simulink model "SOGI_PLL_test"  (R2025a)
settings: Solver=FixedStepAuto  StartTime=0.0  StopTime=0.4  FixedStep=sample_time_s_d  RelTol=1e-3  EnableMultiTasking=on
undefined symbols (not defined in the file): DiscIntNeverNeededParam, filter_omega_sogi_a, filter_omega_sogi_b, filter_omega_sogi_init, filter_rms_out_a, filter_rms_out_b, filter_rms_out_init, grid_frequency_hz, k_rms, k_sogi_5th_hardmonic, pll_sat_max, pll_sat_min, SRF_PI_I, SRF_PI_P, Ts
libraries: simulink x2, spsAlphaBetaZerotodq0Lib x1, eeDiscretePi x1
settings Model: Creator=Masood  LastModifiedBy=li_hh
settings OptimizationCC: DefaultParameterBehavior=Inlined  UseDivisionForNetSlopeComputation=on  GainParamInheritBuiltInType=on  UseFloatMulNetSlope=on  InlineInvariantSignals=on  PassReuseOutputArgsAs=Individual arguments  ZeroExternalMemoryAtStartup=off  NoFixptDivByZeroProtection=on  EfficientFloat2IntCast=on  LifeSpan=1  MaxStackSize=2560  OptimizeBlockOrder=speed  DifferentSizesBufferReuse=on  EfficientTunableParamExpr=on
settings DebuggingCC: ParameterTunabilityLossMsg=error
settings HardwareCC: ProdBitPerPointer=32.0  ProdBitPerSizeT=32.0  ProdBitPerPtrDiffT=32.0  ProdLargestAtomicInteger=Long  ProdLargestAtomicFloat=Double  ProdWordSize=32.0  ProdLongLongMode=on  ProdHWDeviceType=ARM Compatible->ARM Cortex-M
settings SFSimCC: MATLABDynamicMemAlloc=off
settings RTWCC: SystemTargetFile=ert.tlc  TemplateMakefile=ert_default_tmf  Toolchain=Texas Instruments Code Composer Studio (ARM)  Description=Embedded Coder
settings CodeAppCC: ForceParamTrailComments=on  IgnoreCustomStorageClasses=off  OperatorAnnotations=on  SimulinkDataObjDesc=on  SFDataObjDesc=on  CustomSymbolStrGlobalVar=rt$N$M  CustomSymbolStrType=$N$M  CustomSymbolStrFcn=$N$M$F  CustomSymbolStrMacro=$N$M  InsertBlockDesc=on
settings ERTTargetCC: ExtModeTransport=3.0  ERTCustomFileTemplate=example_file_process.tlc  ERTFilePackagingFormat=CompactWithDataFile  IncludeMdlTerminateFcn=off  CombineSignalStateStructs=on  CodeInterfacePackaging=Reusable function  SupportComplex=off  SupportContinuousTime=on

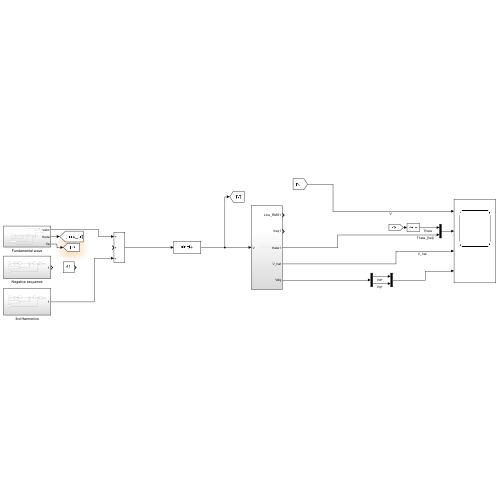
[thumbnail: Simulink's stored preview of the top-level diagram]
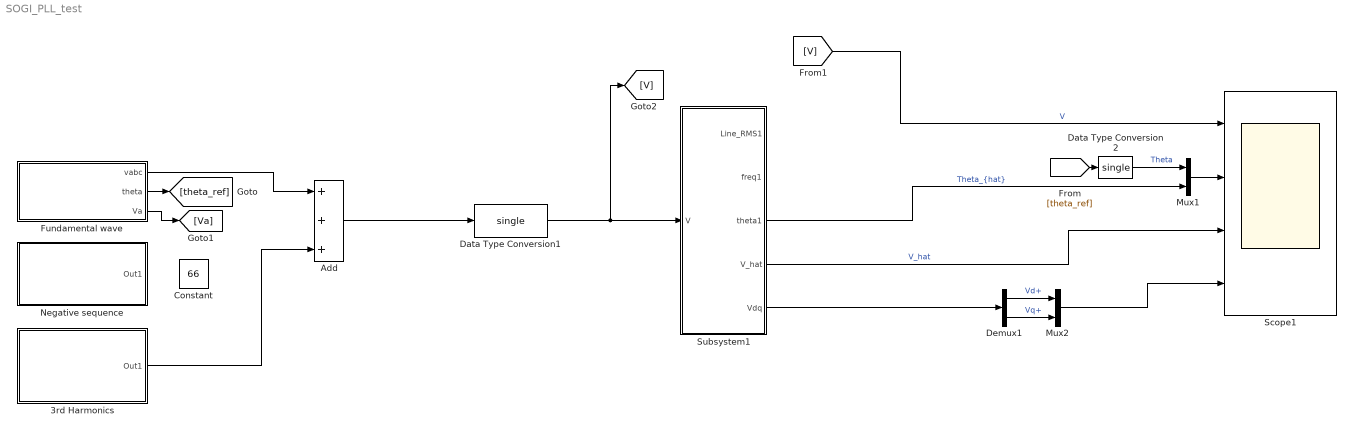
== system SOGI_PLL_test ==
  3rd Harmonics : Subsystem
  Add : Sum  Inputs=+++
  Constant : Constant  Value=66
  Data Type Conversion1 : DataTypeConversion  OutDataTypeStr=single  SaturateOnIntegerOverflow=off  RndMeth=Floor
  Data Type Conversion2 : DataTypeConversion  OutDataTypeStr=single  SaturateOnIntegerOverflow=off  RndMeth=Floor
  Demux1 : Demux  Outputs=2
  Fundamental wave : Subsystem
  Mux1 : Mux  Inputs=2
  Mux2 : Mux  Inputs=2
  Negative sequence : Subsystem
  Scope1 : Scope  NumInputPorts=4
      settings: ActiveDisplayYMinimum=-0.78539812564849831  ActiveDisplayYMaximum=7.0685831308364868  YLabel=Voltage/V
  Subsystem1 : Subsystem
  wires:
  Data Type Conversion1/1 -> [V], Subsystem1/1(V)
  Add/1 -> Data Type Conversion1/1
  Fundamental wave/1(vabc) -> Add/1
  Fundamental wave/3(Va) -> [Va]
  Fundamental wave/2(theta) -> [theta_ref]
  [V] -> Scope1/1  "V"
  Subsystem1/3(theta1) -> Mux1/2  "Theta_{hat}"
  Data Type Conversion2/1 -> Mux1/1  "Theta"
  [theta_ref] -> Data Type Conversion2/1
  Mux1/1 -> Scope1/2
  Subsystem1/4(V_hat) -> Scope1/3  "V_hat"
  Demux1/2 -> Mux2/2  "Vq+"
  Mux2/1 -> Scope1/4
  Demux1/1 -> Mux2/1  "Vd+"
  Subsystem1/5(Vdq) -> Demux1/1
  3rd Harmonics/1(Out1) -> Add/3

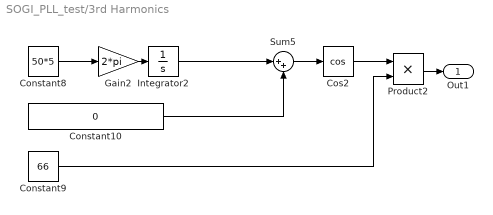
== system SOGI_PLL_test/3rd Harmonics ==
  Constant10 : Constant  Value=0
  Constant8 : Constant  Value=50*5
  Constant9 : Constant  Value=66
  Cos2 : Trigonometry  Operator=cos
  Gain2 : Gain  Gain=2*pi
  Integrator2 : Integrator
  Product2 : Product
  Sum5 : Sum  Inputs=|++
  Out1 : Outport
  wires:
  Constant8/1 -> Gain2/1
  Constant9/1 -> Product2/2
  Cos2/1 -> Product2/1
  Product2/1 -> Out1/1
  Constant10/1 -> Sum5/2
  Integrator2/1 -> Sum5/1
  Gain2/1 -> Integrator2/1
  Sum5/1 -> Cos2/1

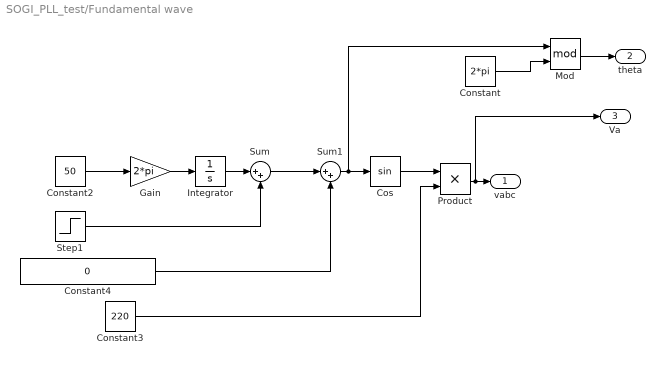
== system SOGI_PLL_test/Fundamental wave ==
  Constant : Constant  Value=2*pi
  Constant2 : Constant  Value=50
  Constant3 : Constant  Value=220
  Constant4 : Constant  Value=0
  Cos : Trigonometry
  Gain : Gain  Gain=2*pi
  Integrator : Integrator
  Mod : Math  Operator=mod
  Product : Product
  Step1 : Step  Time=0.1  After=-pi
  Sum : Sum  Inputs=|++
  Sum1 : Sum  Inputs=|++
  vabc : Outport
  theta : Outport  Port=2
  Va : Outport  Port=3
  wires:
  Step1/1 -> Sum/2
  Cos/1 -> Product/1
  Integrator/1 -> Sum/1
  Constant3/1 -> Product/2
  Constant4/1 -> Sum1/2
  Sum/1 -> Sum1/1
  Constant2/1 -> Gain/1
  Gain/1 -> Integrator/1
  Product/1 -> Va/1, vabc/1
  Mod/1 -> theta/1
  Constant/1 -> Mod/2
  Sum1/1 -> Mod/1, Cos/1

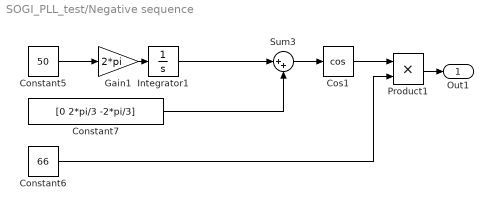
== system SOGI_PLL_test/Negative sequence ==
  Constant5 : Constant  Value=50
  Constant6 : Constant  Value=66
  Constant7 : Constant  Value=[0 2*pi/3 -2*pi/3]
  Cos1 : Trigonometry  Operator=cos
  Gain1 : Gain  Gain=2*pi
  Integrator1 : Integrator
  Product1 : Product
  Sum3 : Sum  Inputs=|++
  Out1 : Outport
  wires:
  Integrator1/1 -> Sum3/1
  Cos1/1 -> Product1/1
  Constant7/1 -> Sum3/2
  Constant6/1 -> Product1/2
  Gain1/1 -> Integrator1/1
  Constant5/1 -> Gain1/1
  Product1/1 -> Out1/1
  Sum3/1 -> Cos1/1

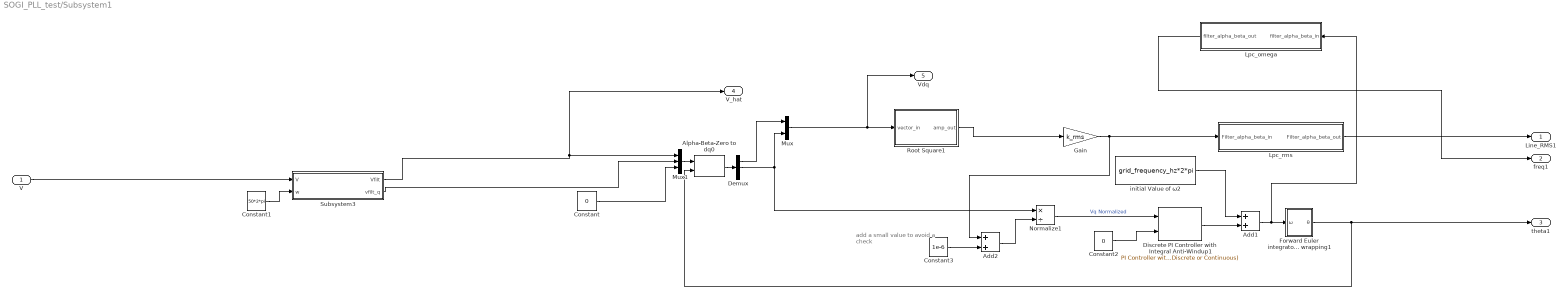
== system SOGI_PLL_test/Subsystem1 ==
  note: add a small value to
      | avoid a check
  V : Inport
  Add1 : Sum
  Add2 : Sum  OutDataTypeStr=single
  Alpha-Beta-Zero to dq0 : spsAlphaBetaZerotodq0Lib/Alpha-Beta-Zero to dq0  Alignment=90 degrees behind phase A axis
  Constant : Constant  Value=0  OutDataTypeStr=single
  Constant1 : Constant  Value=50*2*pi  OutDataTypeStr=single
  Constant2 : Constant  Value=0  OutDataTypeStr=single
  Constant3 : Constant  Value=1e-6  OutDataTypeStr=single
  Demux : Demux  Outputs=3
  Discrete PI Controller with Integral Anti-Windup1 : eeDiscretePi/PI Controller with Integral Anti-Windup (Discrete or Continuous)  Kp=SRF_PI_P  Ki=SRF_PI_I  x0=0  B=pll_sat_max  A=pll_sat_min  Ts=-1
  Forward Euler integrator 2π wrapping1 : Subsystem
  Gain : Gain  Gain=k_rms
  Lpc_omega : Subsystem
  Lpc_rms : Subsystem
  Mux : Mux  Inputs=2
  Mux1 : Mux  Inputs=3
  Normalize1 : Product  Inputs=*/
  Root Square1 : Subsystem
  Subsystem3 : Subsystem
  initial Value of ω2 : Constant  Value=grid_frequency_hz*2*pi  OutDataTypeStr=single
  Line_RMS1 : Outport  OutDataTypeStr=single  PortDimensions=1
  freq1 : Outport  Port=2  OutDataTypeStr=single  PortDimensions=1
  theta1 : Outport  Port=3  OutDataTypeStr=single  PortDimensions=1
  V_hat : Outport  Port=4
  Vdq : Outport  Port=5
  wires:
  Discrete PI Controller with Integral Anti-Windup1/1 -> Add1/2
  Mux/1 -> Vdq/1, Root Square1/1(vector_in)
  Lpc_omega/1(filter_alpha_beta_out) -> freq1/1
  initial Value of ω2/1 -> Add1/1
  Root Square1/1(amp_out) -> Gain/1
  Normalize1/1 -> Discrete PI Controller with Integral Anti-Windup1/1  "Vq Normalized"
  Constant2/1 -> Discrete PI Controller with Integral Anti-Windup1/2
  Demux/2 -> Normalize1/1, Mux/2
  Subsystem3/1(Vfilt) -> Mux1/1, V_hat/1
  Demux/1 -> Mux/1
  Add2/1 -> Normalize1/2
  Constant3/1 -> Add2/2
  Subsystem3/2(vfilt_q) -> Mux1/2
  V/1 -> Subsystem3/1(V)
  Gain/1 -> Add2/1, Lpc_rms/1(Filter_alpha_beta_in)
  Lpc_rms/1(Filter_alpha_beta_out) -> Line_RMS1/1
  Add1/1 -> Lpc_omega/1(filter_alpha_beta_in), Forward Euler integrator 2π wrapping1/1(ω)
  Forward Euler integrator 2π wrapping1/1(θ) -> Alpha-Beta-Zero to dq0/2, theta1/1
  Mux1/1 -> Alpha-Beta-Zero to dq0/1
  Constant/1 -> Mux1/3
  Alpha-Beta-Zero to dq0/1 -> Demux/1
  Constant1/1 -> Subsystem3/2(w)

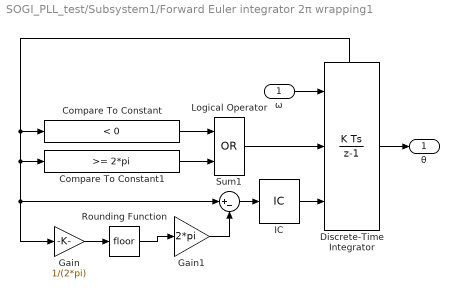
== system SOGI_PLL_test/Subsystem1/Forward Euler integrator 2π wrapping1 ==
  ω : Inport
  Compare To Constant : simulink/Logic and Bit Operations/Compare To Constant  relop=<  const=0  OutDataTypeStr=boolean
  Compare To Constant1 : simulink/Logic and Bit Operations/Compare To Constant  relop=>=  const=2*pi  OutDataTypeStr=boolean
  Discrete-Time Integrator : DiscreteIntegrator  ExternalReset=sampled level  InitialConditionSource=external  SampleTime=-1  OutDataTypeStr=single  ShowStatePort=on  ICPrevOutput=DiscIntNeverNeededParam  ICPrevScaledInput=DiscIntNeverNeededParam
  Gain : Gain  Gain=1/(2*pi)
      settings: AttributesFormatString=%<Gain>
  Gain1 : Gain  Gain=2*pi
  IC : InitialCondition  Value=0
  Logical Operator : Logic  Operator=OR  AllPortsSameDT=off  OutDataTypeStr=boolean
  Rounding Function : Rounding
  Sum1 : Sum  Inputs=|+-
  θ : Outport
  wires:
  Gain1/1 -> Sum1/2
  Gain/1 -> Rounding Function/1
  IC/1 -> Discrete-Time Integrator/3
  Compare To Constant1/1 -> Logical Operator/2
  Discrete-Time Integrator/State -> Compare To Constant1/1, Sum1/1, Gain/1, Compare To Constant/1
  Compare To Constant/1 -> Logical Operator/1
  Logical Operator/1 -> Discrete-Time Integrator/2
  Sum1/1 -> IC/1
  Rounding Function/1 -> Gain1/1
  ω/1 -> Discrete-Time Integrator/1
  Discrete-Time Integrator/1 -> θ/1

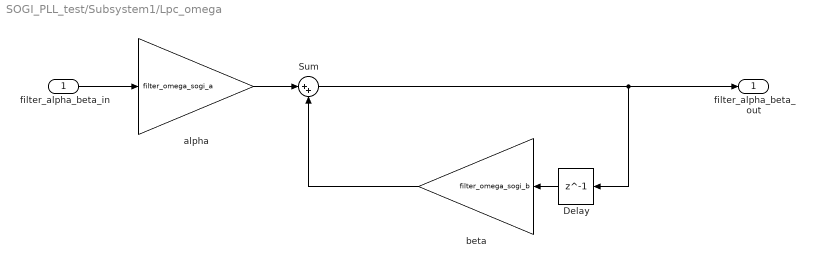
== system SOGI_PLL_test/Subsystem1/Lpc_omega ==
  filter_alpha_beta_in : Inport
  Delay : Delay  DelayLength=1  InitialCondition=filter_omega_sogi_init  InputProcessing=Columns as channels (frame based)
  Sum : Sum  Inputs=|++
  alpha : Gain  Gain=filter_omega_sogi_a
  beta : Gain  Gain=filter_omega_sogi_b
  filter_alpha_beta_out : Outport
  wires:
  Sum/1 -> Delay/1, filter_alpha_beta_out/1
  filter_alpha_beta_in/1 -> alpha/1
  alpha/1 -> Sum/1
  Delay/1 -> beta/1
  beta/1 -> Sum/2

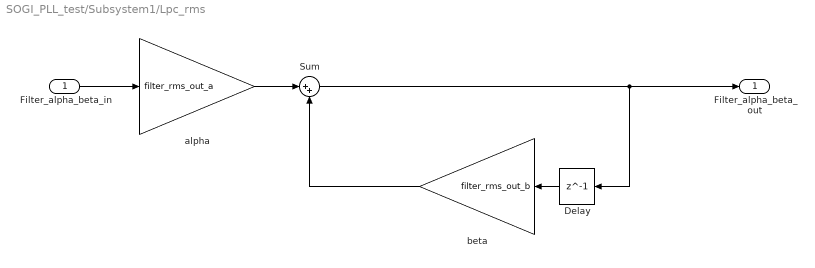
== system SOGI_PLL_test/Subsystem1/Lpc_rms ==
  Filter_alpha_beta_in : Inport
  Delay : Delay  DelayLength=1  InitialCondition=filter_rms_out_init  InputProcessing=Columns as channels (frame based)
  Sum : Sum  Inputs=|++
  alpha : Gain  Gain=filter_rms_out_a
  beta : Gain  Gain=filter_rms_out_b
  Filter_alpha_beta_out : Outport
  wires:
  Sum/1 -> Delay/1, Filter_alpha_beta_out/1
  Filter_alpha_beta_in/1 -> alpha/1
  alpha/1 -> Sum/1
  Delay/1 -> beta/1
  beta/1 -> Sum/2

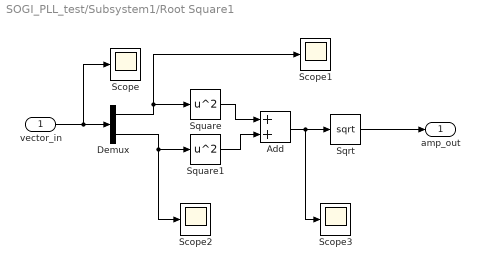
== system SOGI_PLL_test/Subsystem1/Root Square1 ==
  vector_in : Inport
  Add : Sum
  Demux : Demux  Outputs=2
  Scope{,1..3} (4 alike) : Scope
      Scope settings: ActiveDisplayYMinimum=-0.23444  ActiveDisplayYMaximum=1.38688  DataLoggingVariableName=ScopeData7
      Scope1 settings: ActiveDisplayYMinimum=0.75652  ActiveDisplayYMaximum=1.27677  DataLoggingVariableName=ScopeData8
      Scope2 settings: ActiveDisplayYMinimum=-0.19634  ActiveDisplayYMaximum=1.04394  DataLoggingVariableName=ScopeData9
      Scope3 settings: ActiveDisplayYMinimum=-1.24998  ActiveDisplayYMaximum=1.24982  DataLoggingVariableName=ScopeData10
  Sqrt : Sqrt
  Square : Math  Operator=square
  Square1 : Math  Operator=square
  amp_out : Outport
  wires:
  Square/1 -> Add/1
  Add/1 -> Scope3/1, Sqrt/1
  Sqrt/1 -> amp_out/1
  Demux/2 -> Scope2/1, Square1/1
  Square1/1 -> Add/2
  vector_in/1 -> Scope/1, Demux/1
  Demux/1 -> Scope1/1, Square/1

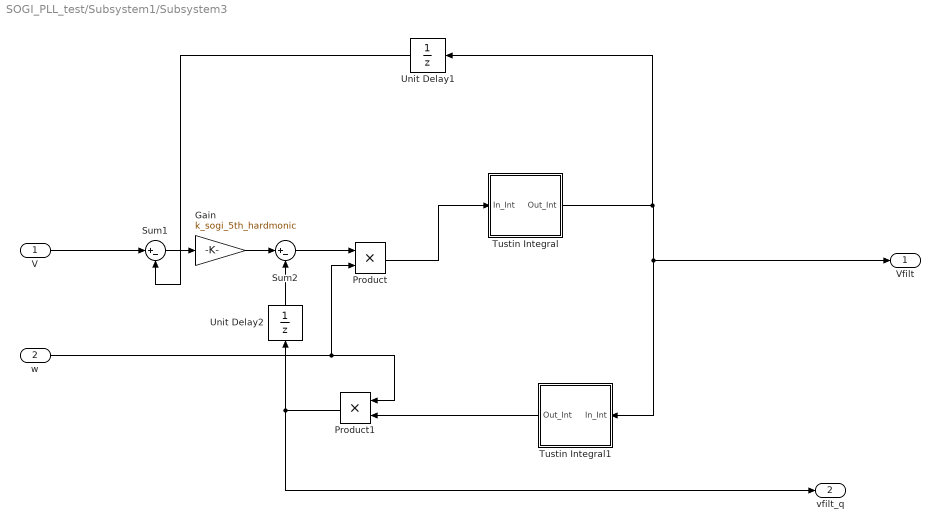
== system SOGI_PLL_test/Subsystem1/Subsystem3 ==
  V : Inport
  w : Inport  Port=2
  Gain : Gain  Gain=k_sogi_5th_hardmonic
  Product : Product
  Product1 : Product
  Sum1 : Sum  Inputs=|+-
  Sum2 : Sum  Inputs=|+-
  Tustin Integral : Subsystem
  Tustin Integral1 : Subsystem
  Unit Delay1 : UnitDelay  SampleTime=-1  HasFrameUpgradeWarning=on
  Unit Delay2 : UnitDelay  SampleTime=-1  HasFrameUpgradeWarning=on
  Vfilt : Outport
  vfilt_q : Outport  Port=2
  wires:
  Unit Delay1/1 -> Sum1/2
  Gain/1 -> Sum2/1
  V/1 -> Sum1/1
  Tustin Integral1/1(Out_Int) -> Product1/2
  Product/1 -> Tustin Integral/1(In_Int)
  Sum1/1 -> Gain/1
  w/1 -> Product/2, Product1/1
  Sum2/1 -> Product/1
  Unit Delay2/1 -> Sum2/2
  Tustin Integral/1(Out_Int) -> Vfilt/1, Tustin Integral1/1(In_Int), Unit Delay1/1
  Product1/1 -> vfilt_q/1, Unit Delay2/1

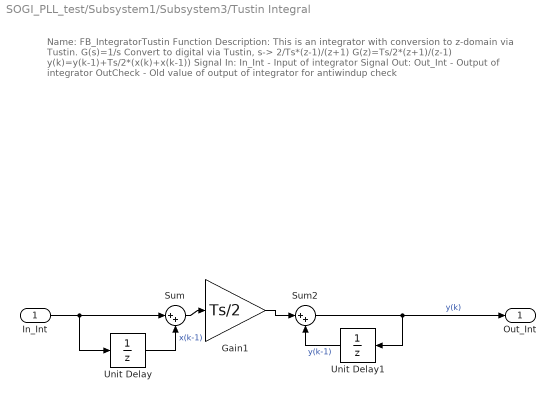
== system SOGI_PLL_test/Subsystem1/Subsystem3/Tustin Integral ==
  note: Name: FB_IntegratorTustin
      |
      | Function Description:
      | This is an integrator with conversion to z-domain via Tustin.
      | G(s)=1/s
      | Convert to digital via Tustin, s-> 2/Ts*(z-1)/(z+1)
      | G(z)=Ts/2*(z+1)/(z-1)
      | y(k)=y(k-1)+Ts/2*(x(k)+x(k-1))
      |
      | Signal In:
      | 	In_Int - Input of integrator
      |
      | Signal Out:
      | 	Out_Int - Output of integrator
      | 	OutCheck - Old value of output of integrator for antiwindup check
  In_Int : Inport
  Gain1 : Gain  Gain=Ts/2
  Sum : Sum  Inputs=|++
  Sum2 : Sum  Inputs=|++
  Unit Delay : UnitDelay  SampleTime=-1  HasFrameUpgradeWarning=on
  Unit Delay1 : UnitDelay  SampleTime=-1  HasFrameUpgradeWarning=on
  Out_Int : Outport
  wires:
  Unit Delay1/1 -> Sum2/2  "y(k-1)"
  Unit Delay/1 -> Sum/2  "x(k-1)"
  In_Int/1 -> Unit Delay/1, Sum/1
  Sum2/1 -> Out_Int/1, Unit Delay1/1  "y(k)"
  Sum/1 -> Gain1/1
  Gain1/1 -> Sum2/1

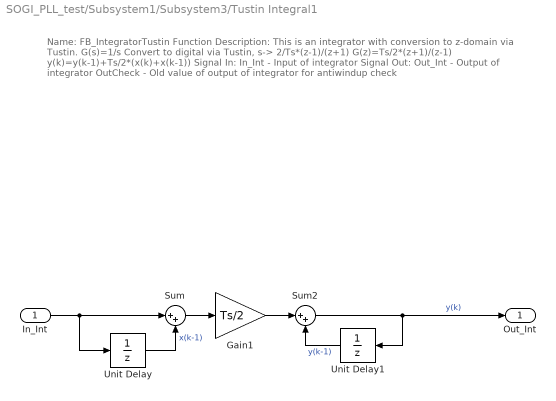
== system SOGI_PLL_test/Subsystem1/Subsystem3/Tustin Integral1 ==
  note: Name: FB_IntegratorTustin
      |
      | Function Description:
      | This is an integrator with conversion to z-domain via Tustin.
      | G(s)=1/s
      | Convert to digital via Tustin, s-> 2/Ts*(z-1)/(z+1)
      | G(z)=Ts/2*(z+1)/(z-1)
      | y(k)=y(k-1)+Ts/2*(x(k)+x(k-1))
      |
      | Signal In:
      | 	In_Int - Input of integrator
      |
      | Signal Out:
      | 	Out_Int - Output of integrator
      | 	OutCheck - Old value of output of integrator for antiwindup check
  In_Int : Inport
  Gain1 : Gain  Gain=Ts/2
  Sum : Sum  Inputs=|++
  Sum2 : Sum  Inputs=|++
  Unit Delay : UnitDelay  SampleTime=-1  HasFrameUpgradeWarning=on
  Unit Delay1 : UnitDelay  SampleTime=-1  HasFrameUpgradeWarning=on
  Out_Int : Outport
  wires:
  Unit Delay1/1 -> Sum2/2  "y(k-1)"
  Unit Delay/1 -> Sum/2  "x(k-1)"
  In_Int/1 -> Unit Delay/1, Sum/1
  Sum2/1 -> Out_Int/1, Unit Delay1/1  "y(k)"
  Sum/1 -> Gain1/1
  Gain1/1 -> Sum2/1
